simulink model "labo1"  (R2018a)
settings: Solver=ode15s  StartTime=0.0  StopTime=0.1  RelTol=1e-3
libraries: powerlib x12, powerlib_meascontrol x1
settings Model: Creator=deniz  LastModifiedBy=deniz

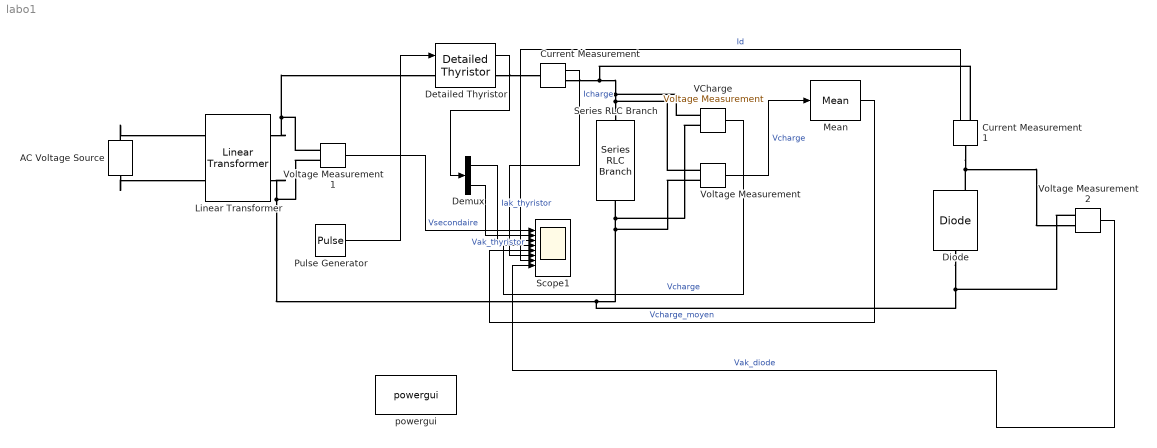
== system labo1 ==
  AC Voltage Source : powerlib/Electrical Sources/AC Voltage Source  Amplitude=170  Phase=0  Frequency=60  SampleTime=0  Measurements=None  BusType=swing  Pref=10e3  Qref=0  Qmin=-inf  Qmax=+inf
  Current Measurement : powerlib/Measurements/Current Measurement  PhasorSimulation=off  OutputType=Complex  PSBequivalent=0
  Current Measurement1 : powerlib/Measurements/Current Measurement  PhasorSimulation=off  OutputType=Complex  PSBequivalent=0
  Demux : Demux  Outputs=2
  Detailed Thyristor : powerlib/Power Electronics/Detailed Thyristor  Ron=0.1  Lon=10e-6  Vf=0.8  IL=0.3  Tq=100e-6  IC=0  Rs=1000  Cs=1e-7  Measurements=on
      settings: SourceProductName=Simscape Power Systems  SourceProductBaseCode=PS
  Diode : powerlib/Power Electronics/Diode  Ron=0.1  Lon=0  Vf=0.8  IC=0  UseSnubber=0  Rs=100  Cs=4e-6  Measurements=on
  Linear Transformer : powerlib/Elements/Linear Transformer  UNITS=pu  NominalPower=[1e3 60]  winding1=[120 0.06944 0.080001]  winding2=[120 0.06944 0.080001]  ThreeWindings=off  winding3=[3.15e+05 0.002 0.079999]  RmLm=[500 500]  Measurements=None  DataType=off
  Mean : powerlib_meascontrol/Measurements/Mean  Freq=60  Vinit=0  Ts=0
  Pulse Generator : DiscretePulseGenerator  PulseType=Time based  Period=1/60  PulseWidth=5  PhaseDelay=(1/60)*(60/360)
  Scope1 : Scope  NumInputPorts=8
  Series RLC Branch : powerlib/Elements/Series RLC Branch  LConnTagsString=__new0  RConnTagsString=__new0  BranchType=RLC  Resistance=10  Inductance=50e-3  SetiL0=off  InitialCurrent=0  Capacitance=inf  Setx0=off  InitialVoltage=0  Measurements=None
  VCharge : powerlib/Measurements/Voltage Measurement  PhasorSimulation=off  OutputType=Complex  PSBequivalent=0
  Voltage Measurement : powerlib/Measurements/Voltage Measurement  PhasorSimulation=off  OutputType=Complex  PSBequivalent=0
  Voltage Measurement1 : powerlib/Measurements/Voltage Measurement  PhasorSimulation=off  OutputType=Complex  PSBequivalent=0
  Voltage Measurement2 : powerlib/Measurements/Voltage Measurement  PhasorSimulation=off  OutputType=Complex  PSBequivalent=0
  powergui : powerlib/powergui  Priority=1  SimulationMode=Continuous  SampleTime=50e-6  frequency=60  Iterations=50  frequencyindice=0  Pbase=100e6  ErrMax=1e-4  UnitsV=kV  UnitsW=MW  buscounter=0  FunctionMessages=off  echomessages=off  EnableUseOfTLC=off  CurrentSourceSwitches=off  DisableSnubberDevices=off  DisableRonSwitches=off  DisableVfSwitches=off  DisplayEquations=off  SolverType=Tustin/Backward Euler (TBE)  Interpol=off  ExternalGateDelay=off  methode=off  Ts=100  x0status=blocks  SPID=off  SwTol=0  HookPort=off  RestoreLinks=warning  ResistiveCurrentMeasurement=off  Frange=[0:2:500]  Ylog=off  Xlog=on  ShowGrid=off  save=off  variable=ZData  structure=0  ZoomFFT=off  StartTime=0.0  cycles=1  DisplayStyle=1  fundamental=60  FreqAxis=off  MaxFrequency=1000  frequencyindicesteady=1  RmsSteady=1  display=off
  wires:
  Pulse Generator/1 -> Detailed Thyristor/1
  Current Measurement/1 -> Scope1/6  "Icharge"
  Detailed Thyristor/1 -> Demux/1
  Demux/2 -> Scope1/2  "Vak_thyristor"
  Voltage Measurement/1 -> Mean/1  "Vcharge"
  Voltage Measurement1/1 -> Scope1/1  "Vsecondaire"
  Mean/1 -> Scope1/5  "Vcharge_moyen"
  VCharge/1 -> Scope1/4  "Vcharge"
  Voltage Measurement2/1 -> Scope1/8  "Vak_diode"
  Demux/1 -> Scope1/3  "Iak_thyristor"
  Current Measurement1/1 -> Scope1/7  "Id"
  connections:
  AC Voltage Source/RConn1 -- Linear Transformer/LConn1
  AC Voltage Source/LConn1 -- Linear Transformer/LConn2
  Linear Transformer/RConn1 -- Voltage Measurement1/LConn1 -- Detailed Thyristor/LConn1
  Detailed Thyristor/RConn1 -- Current Measurement/LConn1
  Diode/RConn1 -- Current Measurement1/LConn1 -- Voltage Measurement2/LConn2
  Linear Transformer/RConn2 -- Voltage Measurement1/LConn2 -- Voltage Measurement2/LConn1 -- Diode/LConn1 -- Voltage Measurement/LConn2 -- VCharge/LConn2 -- Series RLC Branch/RConn1
  Current Measurement/RConn1 -- Current Measurement1/RConn1 -- VCharge/LConn1 -- Voltage Measurement/LConn1 -- Series RLC Branch/LConn1
